simulink model "UDP_Send_Poi_2021b_openloop_joystick_2023"  (R2021b)
settings: Solver=FixedStepDiscrete  StartTime=0.0  StopTime=inf  FixedStep=0.05  RelTol=1e-3  EnableMultiTasking=on
undefined symbols (not defined in the file or in its folder): alpha_b_gain, DiscIntNeverNeededParam, Ts, z_l_gain
libraries: simulink x21, svdutilitieslib x10, raspberrypiNetworklib x2, dspstat3 x1
settings Model: SimulationMode=external  ExtModeTrigDuration=2  Creator=Sesh  LastModifiedBy=n7729
settings SolverCC: PositivePriorityOrder=on
settings OptimizationCC: EnhancedBackFolding=on  PassReuseOutputArgsAs=Individual arguments  ZeroExternalMemoryAtStartup=off  ZeroInternalMemoryAtStartup=off  MaxStackSize=64  OptimizeBlockOrder=speed  DifferentSizesBufferReuse=on  OptimizationCustomize=off  EfficientTunableParamExpr=on
settings DebuggingCC: ParameterTunabilityLossMsg=error  UnderSpecifiedDimensionMsg=warning
settings HardwareCC: ProdBitPerPointer=32  ProdBitPerSizeT=32  ProdBitPerPtrDiffT=32  ProdLargestAtomicInteger=Long  ProdLargestAtomicFloat=Double  ProdWordSize=32  ProdLongLongMode=on  ProdHWDeviceType=ARM Compatible->ARM Cortex
settings RTWCC: Description=Embedded Coder  SystemTargetFile=ert.tlc  HardwareBoard=Raspberry Pi  TLCOptions="-aInlineSetEventsForThisBaseRateFcn=TLC_FALSE -aSuppressMultiTaskScheduler=TLC_FALSE  -aRateBasedStepFcn=0"  TemplateMakefile=ert_default_tmf  Toolchain=GNU GCC Embedded Linux  BuildConfiguration=Faster Runs
settings CodeAppCC: ForceParamTrailComments=on  IgnoreCustomStorageClasses=off  OperatorAnnotations=on  SimulinkDataObjDesc=on  SFDataObjDesc=on  InsertBlockDesc=on
settings ERTTargetCC: SupportContinuousTime=on  SupportVariableSizeSignals=on  ExtMode=on  ExtModeTransport=2  ExtModeStaticAlloc=on  ExtModeMexFile=ext_xcp  ExtModeMexArgs='192.168.0.112' 0 17725  ExtModeIntrfLevel=Level2 - Open

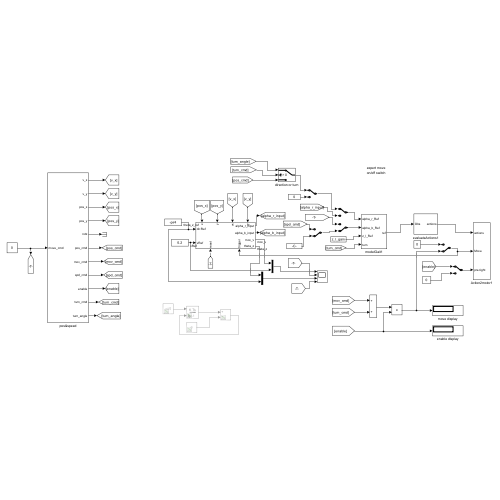
[thumbnail: Simulink's stored preview of the top-level diagram]
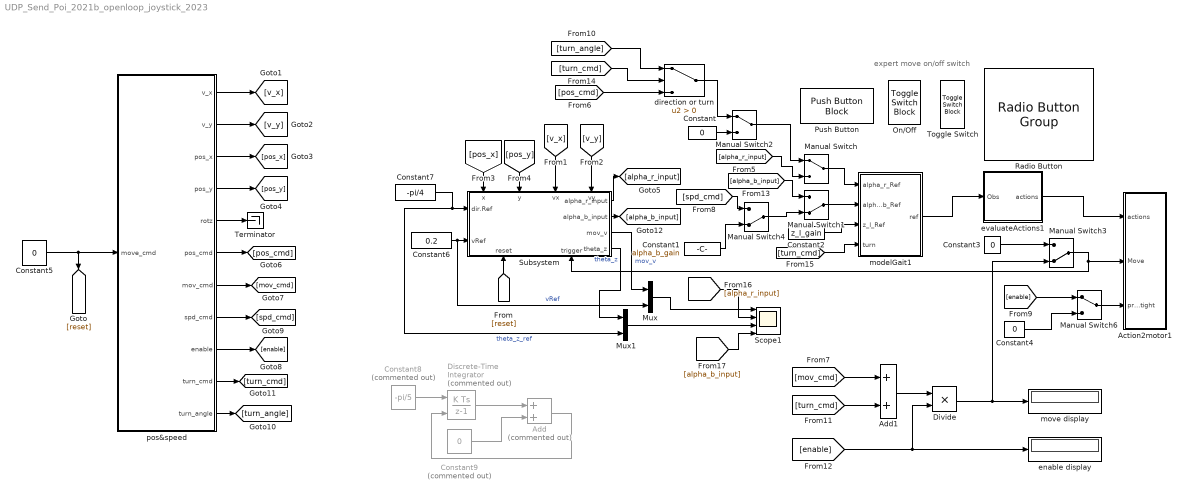
== system UDP_Send_Poi_2021b_openloop_joystick_2023 ==
  note: expert move
      | on/off switch
  Action2motor1 : Subsystem
  Add : Sum  Commented=on
  Add1 : Sum
  Constant{,3..5} (4 alike) : Constant  Value=0
  Constant1 : Constant  Value=alpha_b_gain
  Constant2 : Constant  Value=z_l_gain
  Constant6 : Constant  Value=0.2
  Constant7 : Constant  Value=-pi/4
  Constant8 : Constant  Commented=on  Value=-pi/5
  Constant9 : Constant  Commented=on  Value=0
  Discrete-Time Integrator : DiscreteIntegrator  Commented=on  ExternalReset=falling  SampleTime=Ts  ICPrevOutput=DiscIntNeverNeededParam  ICPrevScaledInput=DiscIntNeverNeededParam
  Divide : Product  Inputs=**
  Manual Switch : ManualSwitch
  Manual Switch1 : ManualSwitch  CurrentSetting=0
  Manual Switch2 : ManualSwitch
  Manual Switch3 : ManualSwitch  CurrentSetting=0
  Manual Switch4 : ManualSwitch  CurrentSetting=0
  Manual Switch6 : ManualSwitch
  Mux : Mux  Inputs=2
  Mux1 : Mux  Inputs=2
  On/Off : ToggleSwitchBlock  LabelPosition=Hide
      settings: Values={{'Off', 'On'}, [0 1]}
  Push Button : PushButtonBlock  ButtonText=reset_pos  OffValue=0.000000
  Radio Button : RadioButtonGroup  LabelPosition=Hide  SelectedLabel=front  ButtonGroupName=Direction
      settings: Values={{'front', 'back', 'left', 'right'}, [0 3.1416 1.5708 -1.5708]}
  Scope1 : Scope  NumInputPorts=4
  Subsystem : Subsystem
      settings: PortSchema="{\"entries\":[{\"content\":{\"sides\":[{\"content\":{\"connectorIds\":[\"In1\",\"In2\"]},\"type\":\"ConnectorPlacement.EquallySpacedRectSide\",\"uuid\":\"e0270cc0-a6da-4fa7-8263-2e1b5ac58467\"},{\"content\":{\"connectorIds\":[\"Out1\",\"Out2\",\"Out3\",\"Out4\"],\"side\":\"RIGHT\"},\"type\":\"ConnectorPlacement.EquallySpacedRectSide\",\"uuid\":\"f8f4d5ad-7603-452d-addd-169a876a6d80\"},{\"content\":{\"connectorIds\":[\"In3\",\"In4\",\"In5\",\"In6\"],\"side\":\"TOP\"},\"type\":\"ConnectorPlacement.EquallySpacedRectSide\",\"uuid\":\"9d841264-c6b3-49f6-8890-3bf3ae488520\"},{\"content\":{\"connectorIds\":[\"In7\",\"In8\"],\"side\":\"BOTTOM\"},\"type\":\"ConnectorPlacement.EquallySpacedRectSide\",\"uuid\":\"4462aa19-ad84-4319-8adf-52b01e042218\"}]},\"type\":\"ConnectorPlacement.EquallySpacedConnector\",\"uuid\":\"62223290-ed65-4858-a6ef-8a0888ac6d95\"}],\"packageUris\":[\"http://schema.mathworks.com/mf0/Connector/R2020b\"],\"version\":\"1.0\"}"
  Terminator : Terminator
  Toggle Switch : ToggleSwitchBlock  LabelPosition=Hide
      settings: Values={{'loose', 'tight'}, [0 1]}
  direction or turn : Switch  Criteria=u2 > Threshold
  enable display : Display
  evaluateActions1 : Subsystem
  modelGait1 : Subsystem
  move display : Display
  pos&speed : Subsystem
  wires:
  [turn_cmd] -> Add1/2
  Discrete-Time Integrator/1 -> Add/1
  Subsystem/2(alpha_b_input) -> [alpha_b_input]
  [alpha_r_input] -> Scope1/2
  Subsystem/1(alpha_r_input) -> [alpha_r_input]
  pos&speed/2(v_y) -> [v_y]
  modelGait1/1(ref) -> evaluateActions1/1(Obs)
  pos&speed/5(rotz) -> Terminator/1
  [mov_cmd] -> Add1/1
  Constant9/1 -> Add/2
  [spd_cmd] -> Manual Switch4/1
  Manual Switch3/1 -> Action2motor1/2(Move), Subsystem/8(trigger)
  pos&speed/9(enable) -> [enable]
  pos&speed/7(mov_cmd) -> [mov_cmd]
  pos&speed/1(v_x) -> [v_x]
  [pos_y] -> Subsystem/4(y)
  [alpha_r_input] -> Manual Switch/2
  [enable] -> Manual Switch6/1
  Subsystem/3(mov_v) -> Mux/1  "mov_v"
  pos&speed/11(turn_angle) -> [turn_angle]
  [pos_cmd] -> direction or turn/3
  [v_x] -> Subsystem/5(vx)
  pos&speed/3(pos_x) -> [pos_x]
  evaluateActions1/1(actions) -> Action2motor1/1(actions)
  Manual Switch1/1 -> modelGait1/2(alpha_b_Ref)
  pos&speed/6(pos_cmd) -> [pos_cmd]
  Constant7/1 -> Mux1/2, Subsystem/1(dir.Ref)  "theta_z_ref"
  [turn_cmd] -> modelGait1/4(turn)
  [v_y] -> Subsystem/6(vy)
  [alpha_b_input] -> Scope1/4
  pos&speed/10(turn_cmd) -> [turn_cmd]
  Divide/1 -> Manual Switch3/2, move display/1
  [turn_cmd] -> direction or turn/2
  Manual Switch4/1 -> Manual Switch1/2
  Constant3/1 -> Manual Switch3/1
  Constant8/1 -> Discrete-Time Integrator/1
  Subsystem/4(theta_z) -> Mux1/1  "theta_z"
  Constant2/1 -> modelGait1/3(z_l_Ref)
  [alpha_b_input] -> Manual Switch1/1
  Constant4/1 -> Manual Switch6/2
  Add1/1 -> Divide/1
  [reset] -> Subsystem/7(reset)
  pos&speed/8(spd_cmd) -> [spd_cmd]
  Manual Switch6/1 -> Action2motor1/3(pre-tight)
  Constant1/1 -> Manual Switch4/2
  Constant/1 -> Manual Switch2/2
  direction or turn/1 -> Manual Switch2/1
  pos&speed/4(pos_y) -> [pos_y]
  Manual Switch/1 -> modelGait1/1(alpha_r_Ref)
  [turn_angle] -> direction or turn/1
  Mux/1 -> Scope1/1
  Add/1 -> Discrete-Time Integrator/2
  [enable] -> enable display/1, Divide/2
  Constant6/1 -> Mux/2, Subsystem/2(vRef)  "vRef"
  Constant5/1 -> [reset], pos&speed/1(move_cmd)
  Mux1/1 -> Scope1/3
  Manual Switch2/1 -> Manual Switch/1
  [pos_x] -> Subsystem/3(x)

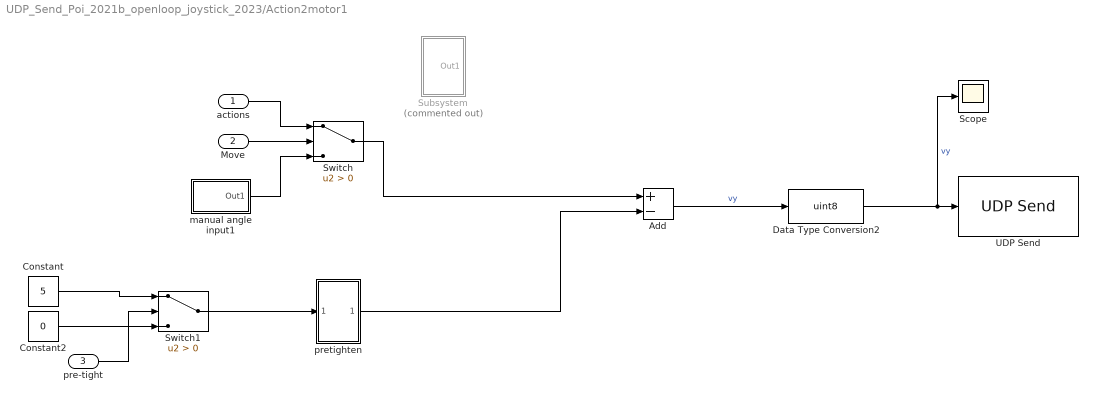
== system UDP_Send_Poi_2021b_openloop_joystick_2023/Action2motor1 ==
  actions : Inport
  Move : Inport  Port=2
  pre-tight : Inport  Port=3
  Add : Sum  Inputs=+-
  Constant : Constant  Value=5
  Constant2 : Constant  Value=0
  Data Type Conversion2 : DataTypeConversion  OutDataTypeStr=uint8
  Scope : Scope
  Subsystem : Subsystem  Commented=on
  Switch : Switch  Criteria=u2 > Threshold
  Switch1 : Switch  Criteria=u2 > Threshold
  UDP Send : raspberrypiNetworklib/UDP Send  remoteURL='0.0.0.0'  remotePort=8888  localURL='0.0.0.0'  localPortSource=Automatically determine  localPort=-1  sampletime=-1  blockPlatform=Raspberry Pi  separateLengthPort=0
      settings: SourceProductBaseCode=RASPPI
  manual angle input1 : Subsystem
  pretighten : Subsystem
  wires:
  actions/1 -> Switch/1
  manual angle input1/1(Out1) -> Switch/3
  pretighten/1(Out1) -> Add/2
  Switch/1 -> Add/1
  Switch1/1 -> pretighten/1(In1)
  Constant/1 -> Switch1/1
  Constant2/1 -> Switch1/3
  Data Type Conversion2/1 -> UDP Send/1, Scope/1  "vy"
  Add/1 -> Data Type Conversion2/1  "vy"
  Move/1 -> Switch/2
  pre-tight/1 -> Switch1/2

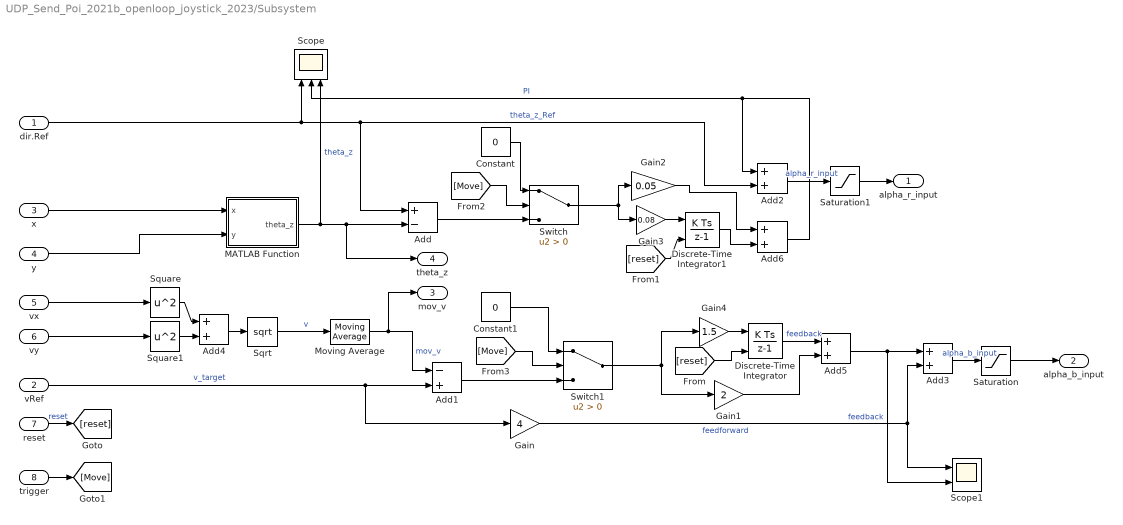
== system UDP_Send_Poi_2021b_openloop_joystick_2023/Subsystem ==
  dir.Ref : Inport
  vRef : Inport  Port=2
  x : Inport  Port=3
  y : Inport  Port=4
  vx : Inport  Port=5
  vy : Inport  Port=6
  reset : Inport  Port=7
  trigger : Inport  Port=8
  Add : Sum  Inputs=+-
  Add1 : Sum  Inputs=-+
  Add{2..6} (5 alike) : Sum
  Constant : Constant  Value=0
  Constant1 : Constant  Value=0
  Discrete-Time Integrator : DiscreteIntegrator  gainval=1  ExternalReset=rising  SampleTime=Ts  ICPrevOutput=DiscIntNeverNeededParam  ICPrevScaledInput=DiscIntNeverNeededParam
  Discrete-Time Integrator1 : DiscreteIntegrator  gainval=1  ExternalReset=rising  SampleTime=-1  ICPrevOutput=DiscIntNeverNeededParam  ICPrevScaledInput=DiscIntNeverNeededParam
  Gain : Gain  Gain=4
  Gain1 : Gain  Gain=2
  Gain2 : Gain  Gain=0.05
  Gain3 : Gain  Gain=0.08
  Gain4 : Gain  Gain=1.5
  MATLAB Function : MATLAB Function  TreatAsAtomicUnit=on
  Moving Average : dspstat3/Moving Average  Method=Sliding window  ForgettingFactorPort=off  SpecifyWindowLength=on  WindowLength=16  ForgettingFactor=0.9  SimulateUsing=Code generation
  Saturation : Saturate  UpperLimit=pi/3  LowerLimit=0
  Saturation1 : Saturate  UpperLimit=inf  LowerLimit=-inf
  Scope : Scope  NumInputPorts=3
  Scope1 : Scope  NumInputPorts=2
  Sqrt : Sqrt  SaturateOnIntegerOverflow=on
  Square : Math  Operator=square  SaturateOnIntegerOverflow=on
  Square1 : Math  Operator=square  SaturateOnIntegerOverflow=on
  Switch : Switch  Criteria=u2 > Threshold
  Switch1 : Switch  Criteria=u2 > Threshold
  alpha_r_input : Outport
  alpha_b_input : Outport  Port=2
  mov_v : Outport  Port=3
  theta_z : Outport  Port=4
  wires:
  Add4/1 -> Sqrt/1
  Square/1 -> Add4/1
  MATLAB Function/1(theta_z) -> Scope/3, Add/2, theta_z/1  "theta_z"
  vRef/1 -> Add1/2, Gain/1  "v_target"
  dir.Ref/1 -> Add2/2, Add/1, Scope/1  "theta_z_Ref"
  Square1/1 -> Add4/2
  Moving Average/1 -> Add1/1, mov_v/1  "mov_v"
  Add6/1 -> Add2/1, Scope/2  "PI"
  Add1/1 -> Switch1/3
  vy/1 -> Square1/1
  Sqrt/1 -> Moving Average/1  "v"
  y/1 -> MATLAB Function/2(y)
  Add2/1 -> Saturation1/1  "alpha_r_input"
  Add3/1 -> Saturation/1  "alpha_b_input"
  x/1 -> MATLAB Function/1(x)
  vx/1 -> Square/1
  Saturation/1 -> alpha_b_input/1
  Saturation1/1 -> alpha_r_input/1
  Switch/1 -> Gain3/1, Gain2/1
  Constant/1 -> Switch/1
  Add/1 -> Switch/3
  Switch1/1 -> Gain1/1, Gain4/1
  Constant1/1 -> Switch1/1
  Discrete-Time Integrator/1 -> Add5/1  "feedback"
  Gain1/1 -> Add5/2
  Discrete-Time Integrator1/1 -> Add6/2
  Gain2/1 -> Add6/1
  Gain3/1 -> Discrete-Time Integrator1/1
  Gain4/1 -> Discrete-Time Integrator/1
  reset/1 -> [reset]  "reset"
  [reset] -> Discrete-Time Integrator/2
  [reset] -> Discrete-Time Integrator1/2
  trigger/1 -> [Move]
  [Move] -> Switch/2
  [Move] -> Switch1/2
  Add5/1 -> Scope1/2, Add3/1  "feedback"
  Gain/1 -> Scope1/1, Add3/2  "feedforward"

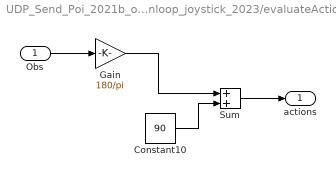
== system UDP_Send_Poi_2021b_openloop_joystick_2023/evaluateActions1 ==
  Obs : Inport
  Constant10 : Constant  Value=90
  Gain : Gain  Gain=180/pi
  Sum : Sum
  actions : Outport  OutDataTypeStr=double
  wires:
  Gain/1 -> Sum/1
  Sum/1 -> actions/1
  Obs/1 -> Gain/1
  Constant10/1 -> Sum/2

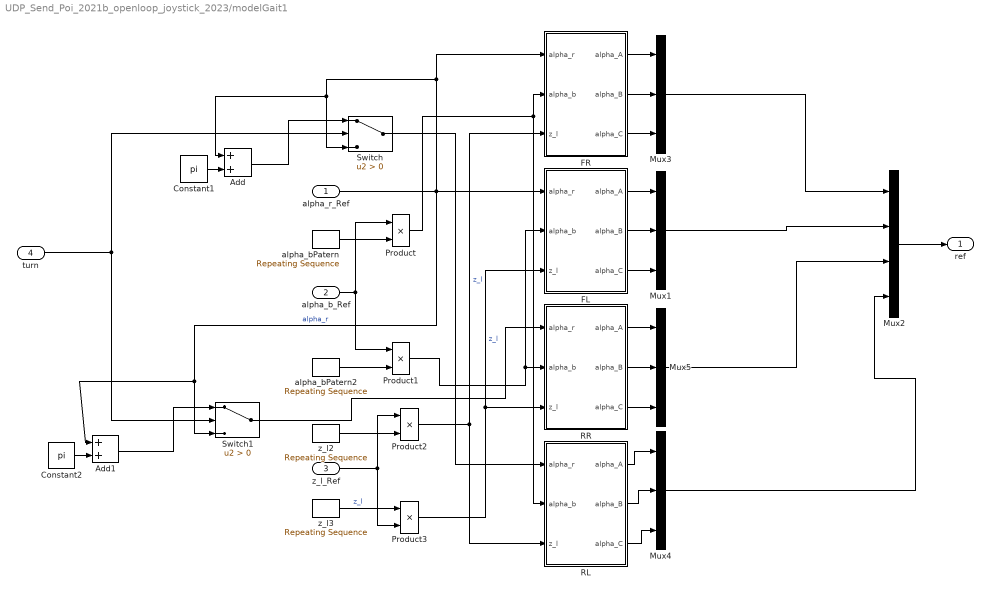
== system UDP_Send_Poi_2021b_openloop_joystick_2023/modelGait1 ==
  alpha_r_Ref : Inport
  alpha_b_Ref : Inport  Port=2
  z_l_Ref : Inport  Port=3
  turn : Inport  Port=4
  Add : Sum
  Add1 : Sum
  Constant1 : Constant  Value=pi
  Constant2 : Constant  Value=pi
  FL : MATLAB Function  TreatAsAtomicUnit=on
  FR : MATLAB Function  TreatAsAtomicUnit=on
  Mux{1,3..5} (4 alike) : Mux  Inputs=3
  Mux2 : Mux
  Product{,1..3} (4 alike) : Product
  RL : MATLAB Function  TreatAsAtomicUnit=on
  RR : MATLAB Function  TreatAsAtomicUnit=on
  Switch : Switch  Criteria=u2 > Threshold
  Switch1 : Switch  Criteria=u2 > Threshold
  alpha_bPatern : simulink/Sources/Repeating Sequence  rep_seq_t=[0 0.2 0.4 0.6 0.8]  rep_seq_y=[0 1 0 -1 0]
  alpha_bPatern2 : simulink/Sources/Repeating Sequence  rep_seq_t=[0 0.2 0.4 0.6 0.8]  rep_seq_y=[0 -1 0 1 0]
  z_l2 : simulink/Sources/Repeating Sequence  rep_seq_t=[0 0.2 0.4 0.6 0.8]  rep_seq_y=[0 0 1 0 0]
  z_l3 : simulink/Sources/Repeating Sequence  rep_seq_t=[0 0.2 0.4 0.6 0.8]  rep_seq_y=[1 0 0 0 1]
  ref : Outport
  wires:
  FR/1(alpha_A) -> Mux3/1
  Product2/1 -> FR/3(z_l), RL/3(z_l)  "z_l"
  FR/2(alpha_B) -> Mux3/2
  FR/3(alpha_C) -> Mux3/3
  Product3/1 -> FL/3(z_l), RR/3(z_l)  "z_l"
  FL/3(alpha_C) -> Mux1/3
  alpha_r_Ref/1 -> Switch1/3, Add1/1, FL/1(alpha_r), FR/1(alpha_r), Switch/3, Add/1  "alpha_r"
  FL/2(alpha_B) -> Mux1/2
  FL/1(alpha_A) -> Mux1/1
  alpha_bPatern/1 -> Product/2
  alpha_b_Ref/1 -> Product/1, Product1/1
  Product/1 -> RL/2(alpha_b), FR/2(alpha_b)
  alpha_bPatern2/1 -> Product1/2
  Product1/1 -> FL/2(alpha_b), RR/2(alpha_b)
  z_l2/1 -> Product2/2
  z_l_Ref/1 -> Product3/2, Product2/1
  z_l3/1 -> Product3/1  "z_l"
  RL/3(alpha_C) -> Mux4/3
  RL/2(alpha_B) -> Mux4/2
  RL/1(alpha_A) -> Mux4/1
  Mux3/1 -> Mux2/1
  RR/3(alpha_C) -> Mux5/3
  RR/1(alpha_A) -> Mux5/1
  RR/2(alpha_B) -> Mux5/2
  Switch/1 -> RL/1(alpha_r)
  Constant1/1 -> Add/2
  Add/1 -> Switch/1
  Switch1/1 -> RR/1(alpha_r)
  Add1/1 -> Switch1/1
  Constant2/1 -> Add1/2
  turn/1 -> Switch1/2, Switch/2
  Mux2/1 -> ref/1
  Mux1/1 -> Mux2/2
  Mux4/1 -> Mux2/4
  Mux5/1 -> Mux2/3

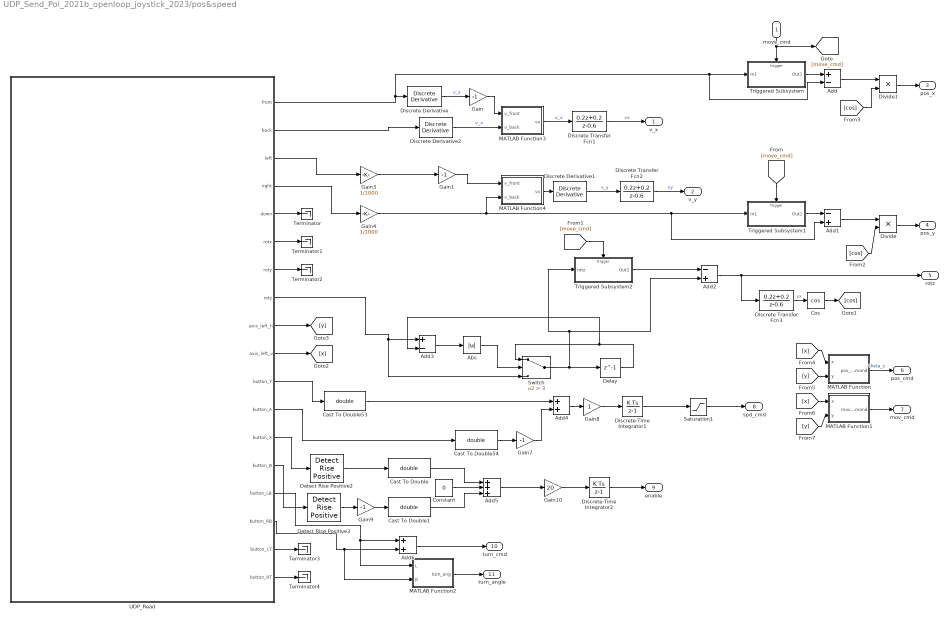
== system UDP_Send_Poi_2021b_openloop_joystick_2023/pos&speed ==
  move_cmd : Inport
  Abs : Abs
  Add : Sum  Inputs=+-
  Add1 : Sum  Inputs=-+
  Add2 : Sum  Inputs=-+
  Add3 : Sum  Inputs=+-
  Add4 : Sum
  Add5 : Sum  Inputs=+++
  Add6 : Sum
  Cast To Double{,1,53..54} (4 alike) : DataTypeConversion  OutDataTypeStr=double
  Constant : Constant  Value=0
  Cos : Trigonometry  Operator=cos
  Delay : Delay  DelayLength=1
  Detect Rise Positive2 : simulink/Logic and Bit Operations/Detect Rise Positive  vinit=0  OutDataTypeStr=boolean
  Detect Rise Positive3 : simulink/Logic and Bit Operations/Detect Rise Positive  vinit=0  OutDataTypeStr=boolean
  Discrete Transfer Fcn1 : DiscreteTransferFcn  Numerator=[0.2 0.2]  Denominator=[1 -0.6]
  Discrete Transfer Fcn2 : DiscreteTransferFcn  Numerator=[0.2 0.2]  Denominator=[1 -0.6]
  Discrete Transfer Fcn3 : DiscreteTransferFcn  Numerator=[0.2 0.2]  Denominator=[1 -0.6]
  Discrete Derivative : simulink/Discrete/Discrete Derivative  gainval=1.0  ICPrevScaledInput=0.0  OutMin=[]  OutMax=[]  OutDataType=fixdt(1, 16)  OutScaling=2^-10  DoSatur=off
  Discrete Derivative1 : simulink/Discrete/Discrete Derivative  gainval=1.0  ICPrevScaledInput=0.0  OutMin=[]  OutMax=[]  OutDataType=fixdt(1, 16)  OutScaling=2^-10  DoSatur=off
  Discrete Derivative2 : simulink/Discrete/Discrete Derivative  gainval=1.0  ICPrevScaledInput=0.0  OutMin=[]  OutMax=[]  OutDataType=fixdt(1, 16)  OutScaling=2^-10  DoSatur=off
  Discrete-Time Integrator1 : DiscreteIntegrator  InitialCondition=pi/12  SampleTime=-1  LimitOutput=on  UpperSaturationLimit=pi/4  LowerSaturationLimit=pi/12  ICPrevOutput=DiscIntNeverNeededParam  ICPrevScaledInput=DiscIntNeverNeededParam
  Discrete-Time Integrator2 : DiscreteIntegrator  SampleTime=-1  LimitOutput=on  UpperSaturationLimit=1  LowerSaturationLimit=0  ICPrevOutput=DiscIntNeverNeededParam  ICPrevScaledInput=DiscIntNeverNeededParam
  Divide : Product  Inputs=**
  Divide1 : Product  Inputs=**
  Gain{,1,7,9} (4 alike) : Gain  Gain=-1
  Gain10 : Gain  Gain=20
  Gain3 : Gain  Gain=1/1000
  Gain4 : Gain  Gain=1/1000
  Gain8 : Gain
  MATLAB Function : MATLAB Function  TreatAsAtomicUnit=on
  MATLAB Function1 : MATLAB Function  TreatAsAtomicUnit=on
  MATLAB Function2 : MATLAB Function  TreatAsAtomicUnit=on
  MATLAB Function3 : MATLAB Function  TreatAsAtomicUnit=on
  MATLAB Function4 : MATLAB Function  TreatAsAtomicUnit=on
  Saturation1 : Saturate  UpperLimit=pi/4  LowerLimit=pi/12
  Switch : Switch  Criteria=u2 > Threshold  Threshold=3
  Terminator{,1..4} (5 alike) : Terminator
  Triggered Subsystem : Subsystem  TreatAsAtomicUnit=on
  Triggered Subsystem1 : Subsystem  TreatAsAtomicUnit=on
  Triggered Subsystem2 : Subsystem  TreatAsAtomicUnit=on
  UDP_Read : Subsystem
  v_x : Outport
  v_y : Outport  Port=2
  pos_x : Outport  Port=3
  pos_y : Outport  Port=4
  rotz : Outport  Port=5
  pos_cmd : Outport  Port=6
  mov_cmd : Outport  Port=7
  spd_cmd : Outport  Port=8
  enable : Outport  Port=9
  turn_cmd : Outport  Port=10
  turn_angle : Outport  Port=11
  wires:
  Gain1/1 -> MATLAB Function4/1(v_front)
  UDP_Read/4(right) -> Gain4/1
  UDP_Read/1(front) -> Discrete Derivative/1, Triggered Subsystem/1(In1), Add/2
  Gain/1 -> MATLAB Function3/1(v_front)
  Gain3/1 -> Gain1/1
  UDP_Read/5(down) -> Terminator/1
  Discrete Derivative1/1 -> Discrete Transfer Fcn2/1  "v_y"
  move_cmd/1 -> Triggered Subsystem/Trigger, [move_cmd]
  Triggered Subsystem/1(Out1) -> Add/1
  Triggered Subsystem1/1(Out1) -> Add1/1
  MATLAB Function4/1(vx) -> Discrete Derivative1/1
  UDP_Read/3(left) -> Gain3/1
  UDP_Read/6(rotx) -> Terminator1/1
  UDP_Read/7(roty) -> Terminator2/1
  Triggered Subsystem2/1(Out1) -> Add2/1
  Add2/1 -> rotz/1, Discrete Transfer Fcn3/1
  Add1/1 -> Divide/1
  Divide/1 -> pos_y/1
  Divide1/1 -> pos_x/1
  Add/1 -> Divide1/1
  Gain4/1 -> MATLAB Function4/2(v_back), Add1/2, Triggered Subsystem1/1(In1)
  Discrete Transfer Fcn1/1 -> v_x/1  "vx"
  Discrete Transfer Fcn2/1 -> v_y/1  "vy"
  Discrete Transfer Fcn3/1 -> Cos/1  "vx"
  UDP_Read/8(rotz) -> Switch/3, Add3/1
  Add3/1 -> Abs/1
  Abs/1 -> Switch/2
  Switch/1 -> Triggered Subsystem2/1(rotz), Add2/2, Delay/1
  Delay/1 -> Add3/2, Switch/1
  MATLAB Function/1(pos_command) -> pos_cmd/1  "theta_z"
  MATLAB Function1/1(move_command) -> mov_cmd/1
  Gain8/1 -> Discrete-Time Integrator1/1
  Discrete-Time Integrator1/1 -> Saturation1/1
  Cast To Double53/1 -> Add4/1
  Gain7/1 -> Add4/2
  UDP_Read/12(button_A) -> Cast To Double54/1
  Add4/1 -> Gain8/1
  Cast To Double54/1 -> Gain7/1
  Saturation1/1 -> spd_cmd/1
  UDP_Read/13(button_X) -> Detect Rise Positive2/1
  UDP_Read/14(button_B) -> Detect Rise Positive3/1
  Detect Rise Positive3/1 -> Gain9/1
  Detect Rise Positive2/1 -> Cast To Double/1
  Gain9/1 -> Cast To Double1/1
  Add5/1 -> Gain10/1
  Discrete-Time Integrator2/1 -> enable/1
  Cast To Double/1 -> Add5/1
  UDP_Read/11(button_Y) -> Cast To Double53/1
  Gain10/1 -> Discrete-Time Integrator2/1
  UDP_Read/15(button_LB) -> MATLAB Function2/1(L), Add6/1
  UDP_Read/16(button_RB) -> MATLAB Function2/2(R), Add6/2
  Add6/1 -> turn_cmd/1
  MATLAB Function2/1(turn_ang) -> turn_angle/1
  [move_cmd] -> Triggered Subsystem1/Trigger
  [move_cmd] -> Triggered Subsystem2/Trigger
  Cos/1 -> [cos]
  [cos] -> Divide1/2
  [cos] -> Divide/2
  UDP_Read/9(axis_left_h) -> [y]
  [x] -> MATLAB Function/1(x)
  [x] -> MATLAB Function1/1(x)
  UDP_Read/10(axis_left_v) -> [x]
  [y] -> MATLAB Function1/2(y)
  [y] -> MATLAB Function/2(y)
  Constant/1 -> Add5/2
  Cast To Double1/1 -> Add5/3
  UDP_Read/17(button_LT) -> Terminator3/1
  UDP_Read/18(button_RT) -> Terminator4/1
  Discrete Derivative/1 -> Gain/1  "v_x"
  Discrete Derivative2/1 -> MATLAB Function3/2(v_back)  "v_x"
  MATLAB Function3/1(vx) -> Discrete Transfer Fcn1/1  "v_x"
  UDP_Read/2(back) -> Discrete Derivative2/1

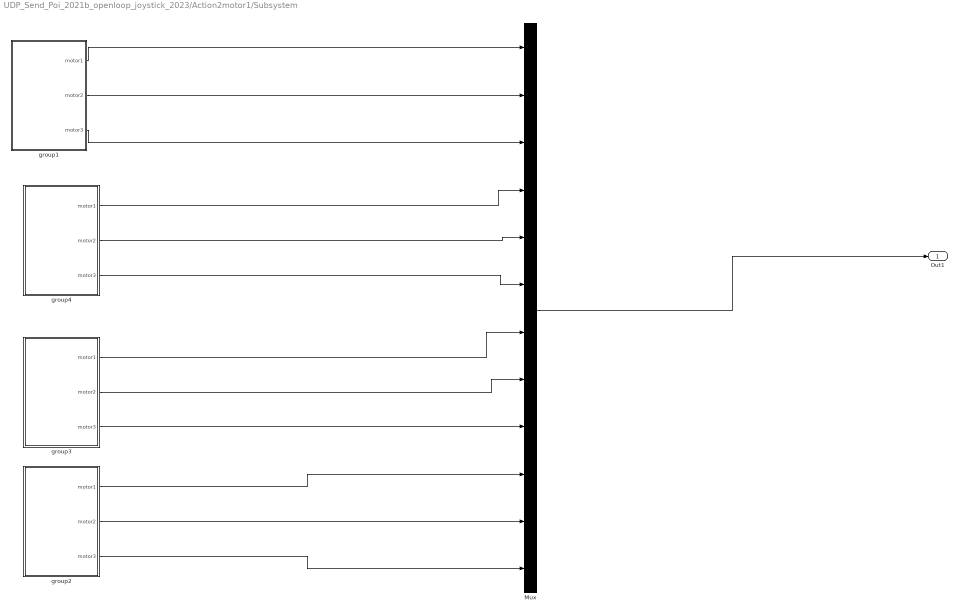
== system UDP_Send_Poi_2021b_openloop_joystick_2023/Action2motor1/Subsystem ==
  Mux : Mux  Inputs=12
  group1 : Subsystem
  group2 : Subsystem
  group3 : Subsystem
  group4 : Subsystem
  Out1 : Outport
  wires:
  group1/1(motor1) -> Mux/1
  group2/1(motor1) -> Mux/10
  group2/3(motor3) -> Mux/12
  group4/2(motor2) -> Mux/5
  group3/2(motor2) -> Mux/8
  group4/1(motor1) -> Mux/4
  group1/3(motor3) -> Mux/3
  group2/2(motor2) -> Mux/11
  group1/2(motor2) -> Mux/2
  Mux/1 -> Out1/1
  group3/1(motor1) -> Mux/7
  group3/3(motor3) -> Mux/9
  group4/3(motor3) -> Mux/6

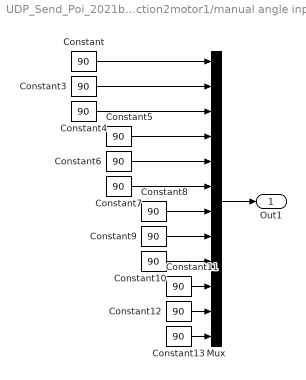
== system UDP_Send_Poi_2021b_openloop_joystick_2023/Action2motor1/manual angle input1 ==
  Constant{,3..13} (12 alike) : Constant  Value=90  SampleTime=-1
  Mux : Mux  Inputs=12
  Out1 : Outport
  wires:
  Constant3/1 -> Mux/2
  Constant11/1 -> Mux/10
  Constant9/1 -> Mux/8
  Constant8/1 -> Mux/7
  Constant/1 -> Mux/1
  Constant4/1 -> Mux/3
  Constant10/1 -> Mux/9
  Constant5/1 -> Mux/4
  Constant7/1 -> Mux/6
  Constant13/1 -> Mux/12
  Constant12/1 -> Mux/11
  Constant6/1 -> Mux/5
  Mux/1 -> Out1/1

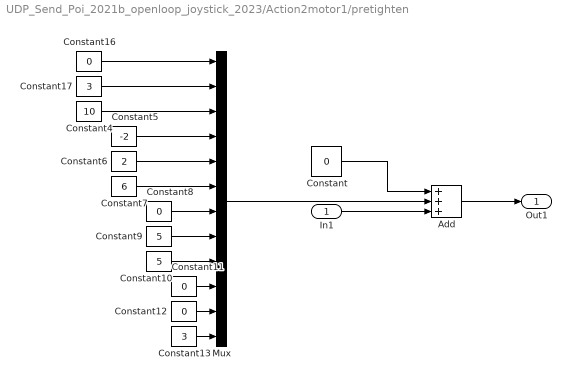
== system UDP_Send_Poi_2021b_openloop_joystick_2023/Action2motor1/pretighten ==
  In1 : Inport
  Add : Sum  Inputs=+++
  Constant : Constant  Value=0
  Constant10 : Constant  Value=5  SampleTime=-1
  Constant{8,11..12,16} (4 alike) : Constant  Value=0  SampleTime=-1
  Constant13 : Constant  Value=3  SampleTime=-1
  Constant17 : Constant  Value=3  SampleTime=-1
  Constant4 : Constant  Value=10  SampleTime=-1
  Constant5 : Constant  Value=-2  SampleTime=-1
  Constant6 : Constant  Value=2  SampleTime=-1
  Constant7 : Constant  Value=6  SampleTime=-1
  Constant9 : Constant  Value=5  SampleTime=-1
  Mux : Mux  Inputs=12
  Out1 : Outport
  wires:
  Constant12/1 -> Mux/11
  Constant6/1 -> Mux/5
  Constant9/1 -> Mux/8
  Constant4/1 -> Mux/3
  Constant13/1 -> Mux/12
  Constant7/1 -> Mux/6
  Constant5/1 -> Mux/4
  Mux/1 -> Add/2
  Constant10/1 -> Mux/9
  Constant8/1 -> Mux/7
  Constant11/1 -> Mux/10
  Constant17/1 -> Mux/2
  Constant/1 -> Add/1
  Constant16/1 -> Mux/1
  Add/1 -> Out1/1
  In1/1 -> Add/3

== system UDP_Send_Poi_2021b_openloop_joystick_2023/pos&speed/Triggered Subsystem ==
  In1 : Inport
  Trigger : TriggerPort  VariantControl=(inherit)
  Out1 : Outport
  wires:
  In1/1 -> Out1/1

== system UDP_Send_Poi_2021b_openloop_joystick_2023/pos&speed/Triggered Subsystem1 ==
  In1 : Inport
  Trigger : TriggerPort  VariantControl=(inherit)
  Out1 : Outport
  wires:
  In1/1 -> Out1/1

== system UDP_Send_Poi_2021b_openloop_joystick_2023/pos&speed/Triggered Subsystem2 ==
  rotz : Inport
  Trigger : TriggerPort  VariantControl=(inherit)
  Out1 : Outport
  wires:
  rotz/1 -> Out1/1

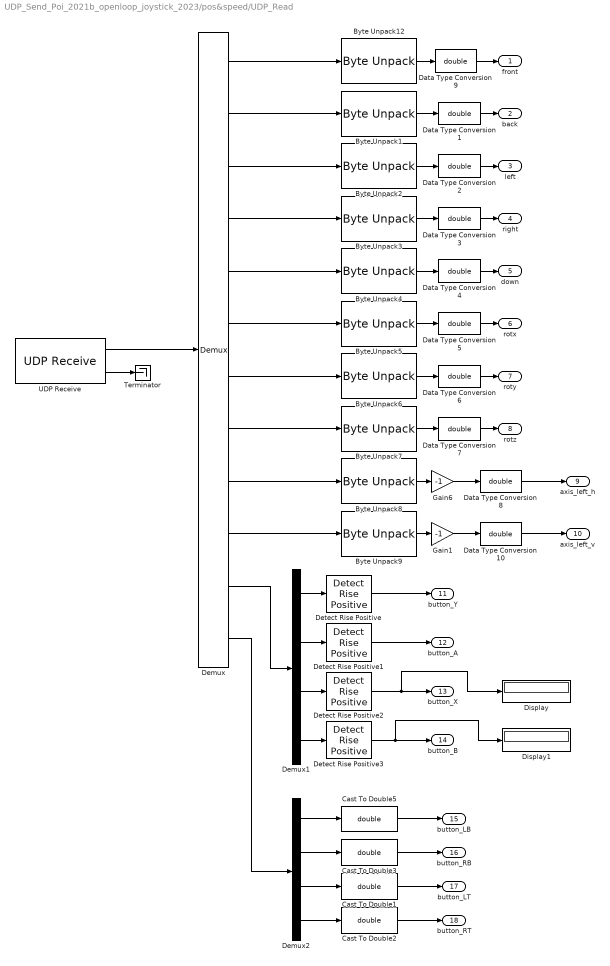
== system UDP_Send_Poi_2021b_openloop_joystick_2023/pos&speed/UDP_Read ==
  Byte Unpack{1..9,12} (10 alike) : svdutilitieslib/Byte Unpack  dimensions={[1]}  datatypes={'single'}  byteAlign=1  blockPlatform=arduinoert
      settings: SourceProductBaseCode=ANDROID,ARDUINO,ML_ARDUINO,ECCORTEXA,ECCORTEXR,SC_BEAGLEBONE_BLUE,EC_FREEDOM_BOARD,EC_FRDM_K64F,INTEL_BLOCKSET,MICROBIT,NUCLEO,NVIDIA,PX4AUTOPILOTS,RASPPIIO,STMICRODIS,TIC2000,XILINX_BLOCKSET
  Cast To Double{1..3,5} (4 alike) : DataTypeConversion  OutDataTypeStr=double
  Data Type Conversion{1..10} (10 alike) : DataTypeConversion  OutDataTypeStr=double
  Demux : Demux  Outputs=12
  Demux1 : Demux
  Demux2 : Demux
  Detect Rise Positive{,1..3} (4 alike) : simulink/Logic and Bit Operations/Detect Rise Positive  vinit=0  OutDataTypeStr=boolean
  Display : Display
  Display1 : Display
  Gain1 : Gain  Gain=-1
  Gain6 : Gain  Gain=-1
  Terminator : Terminator
  UDP Receive : raspberrypiNetworklib/UDP Receive  localURL='0.0.0.0'  localPort=6666  remoteURL='0.0.0.0'  remotePort=-1  recvBufferSize=8192  signalDatatype=uint8  dims=48  isVarSize=off  showBlockingTime=off  blockingTime=0  sampletime=-1  blockPlatform=Raspberry Pi
      settings: SourceProductBaseCode=RASPPI
  front : Outport
  back : Outport  Port=2
  left : Outport  Port=3
  right : Outport  Port=4
  down : Outport  Port=5
  rotx : Outport  Port=6
  roty : Outport  Port=7
  rotz : Outport  Port=8
  axis_left_h : Outport  Port=9
  axis_left_v : Outport  Port=10
  button_Y : Outport  Port=11
  button_A : Outport  Port=12
  button_X : Outport  Port=13
  button_B : Outport  Port=14
  button_LB : Outport  Port=15
  button_RB : Outport  Port=16
  button_LT : Outport  Port=17
  button_RT : Outport  Port=18
  wires:
  Byte Unpack3/1 -> Data Type Conversion3/1
  Byte Unpack12/1 -> Data Type Conversion9/1
  Demux/3 -> Byte Unpack2/1
  Demux/2 -> Byte Unpack1/1
  Demux/5 -> Byte Unpack4/1
  UDP Receive/2 -> Terminator/1
  Byte Unpack4/1 -> Data Type Conversion4/1
  Demux/1 -> Byte Unpack12/1
  Byte Unpack1/1 -> Data Type Conversion1/1
  Byte Unpack2/1 -> Data Type Conversion2/1
  Demux/4 -> Byte Unpack3/1
  Demux/6 -> Byte Unpack5/1
  Demux/7 -> Byte Unpack6/1
  Demux/8 -> Byte Unpack7/1
  Byte Unpack5/1 -> Data Type Conversion5/1
  Byte Unpack6/1 -> Data Type Conversion6/1
  Byte Unpack7/1 -> Data Type Conversion7/1
  Demux/9 -> Byte Unpack8/1
  Demux/10 -> Byte Unpack9/1
  Byte Unpack8/1 -> Gain6/1
  Byte Unpack9/1 -> Gain1/1
  Detect Rise Positive/1 -> button_Y/1
  Demux1/2 -> Detect Rise Positive1/1
  Demux1/3 -> Detect Rise Positive2/1
  Demux1/4 -> Detect Rise Positive3/1
  Demux/11 -> Demux1/1
  Demux1/1 -> Detect Rise Positive/1
  Demux2/1 -> Cast To Double5/1
  Demux2/3 -> Cast To Double1/1
  Demux/12 -> Demux2/1
  Demux2/2 -> Cast To Double3/1
  Demux2/4 -> Cast To Double2/1
  Cast To Double5/1 -> button_LB/1
  Cast To Double3/1 -> button_RB/1
  Data Type Conversion9/1 -> front/1
  Data Type Conversion1/1 -> back/1
  Data Type Conversion2/1 -> left/1
  Data Type Conversion3/1 -> right/1
  Data Type Conversion4/1 -> down/1
  Data Type Conversion5/1 -> rotx/1
  Data Type Conversion6/1 -> roty/1
  Data Type Conversion7/1 -> rotz/1
  Gain6/1 -> Data Type Conversion8/1
  Gain1/1 -> Data Type Conversion10/1
  Data Type Conversion8/1 -> axis_left_h/1
  Data Type Conversion10/1 -> axis_left_v/1
  Detect Rise Positive1/1 -> button_A/1
  Detect Rise Positive2/1 -> Display/1, button_X/1
  Detect Rise Positive3/1 -> Display1/1, button_B/1
  Cast To Double1/1 -> button_LT/1
  Cast To Double2/1 -> button_RT/1
  UDP Receive/1 -> Demux/1

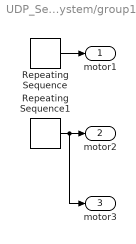
== system UDP_Send_Poi_2021b_openloop_joystick_2023/Action2motor1/Subsystem/group1 ==
  Repeating Sequence : simulink/Sources/Repeating Sequence  rep_seq_t=out.G1M1Data.time  rep_seq_y=out.G1M1Data.signals.values
  Repeating Sequence1 : simulink/Sources/Repeating Sequence  rep_seq_t=out.G1M23Data.time  rep_seq_y=out.G1M23Data.signals.values
  motor1 : Outport  VectorParamsAs1DForOutWhenUnconnected=off
  motor2 : Outport  Port=2  VectorParamsAs1DForOutWhenUnconnected=off
  motor3 : Outport  Port=3  VectorParamsAs1DForOutWhenUnconnected=off
  wires:
  Repeating Sequence1/1 -> motor3/1, motor2/1
  Repeating Sequence/1 -> motor1/1

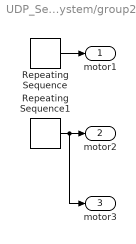
== system UDP_Send_Poi_2021b_openloop_joystick_2023/Action2motor1/Subsystem/group2 ==
  Repeating Sequence : simulink/Sources/Repeating Sequence  rep_seq_t=out.G1M1Data.time  rep_seq_y=out.G1M1Data.signals.values
  Repeating Sequence1 : simulink/Sources/Repeating Sequence  rep_seq_t=out.G1M23Data.time  rep_seq_y=out.G1M23Data.signals.values
  motor1 : Outport  VectorParamsAs1DForOutWhenUnconnected=off
  motor2 : Outport  Port=2  VectorParamsAs1DForOutWhenUnconnected=off
  motor3 : Outport  Port=3  VectorParamsAs1DForOutWhenUnconnected=off
  wires:
  Repeating Sequence1/1 -> motor3/1, motor2/1
  Repeating Sequence/1 -> motor1/1

== system UDP_Send_Poi_2021b_openloop_joystick_2023/Action2motor1/Subsystem/group3 ==
  Repeating Sequence : simulink/Sources/Repeating Sequence  rep_seq_t=out.G3M1Data1.time  rep_seq_y=out.G3M1Data1.signals.values
  Repeating Sequence1 : simulink/Sources/Repeating Sequence  rep_seq_t=out.G3M23Data.time  rep_seq_y=out.G3M23Data.signals.values
  motor1 : Outport  VectorParamsAs1DForOutWhenUnconnected=off
  motor2 : Outport  Port=2  VectorParamsAs1DForOutWhenUnconnected=off
  motor3 : Outport  Port=3  VectorParamsAs1DForOutWhenUnconnected=off
  wires:
  Repeating Sequence1/1 -> motor3/1, motor2/1
  Repeating Sequence/1 -> motor1/1

== system UDP_Send_Poi_2021b_openloop_joystick_2023/Action2motor1/Subsystem/group4 ==
  Repeating Sequence : simulink/Sources/Repeating Sequence  rep_seq_t=out.G3M1Data1.time  rep_seq_y=out.G3M1Data1.signals.values
  Repeating Sequence1 : simulink/Sources/Repeating Sequence  rep_seq_t=out.G3M23Data.time  rep_seq_y=out.G3M23Data.signals.values
  motor1 : Outport  VectorParamsAs1DForOutWhenUnconnected=off
  motor2 : Outport  Port=2  VectorParamsAs1DForOutWhenUnconnected=off
  motor3 : Outport  Port=3  VectorParamsAs1DForOutWhenUnconnected=off
  wires:
  Repeating Sequence1/1 -> motor3/1, motor2/1
  Repeating Sequence/1 -> motor1/1

== matlab function UDP_Send_Poi_2021b_openloop_joystick_2023/pos&speed/MATLAB Function ==
  data: x input; pos_command output; y input
function pos_command = fcn(x, y)
if y >=-0.5 && y<= 0.5 && x >= -0.5 && x <= 0.5
    pos_command = 0; % no move, joystick in center
else
if y == 0 && x >= 0
    pos_command = 0; % joystick up, move forward
elseif y == 0 && x < 0
    pos_command = pi; % joystick down, move backward
else
    pos_command = atan(y/x); % o.w., calculate the turn angle
end

% limit the angle calculation
if x<0 && y<0
    pos_command = pos_command - pi;
end
if x<0 && y>0
    pos_command = pos_command + pi;
end

if pos_command < -pi*0.99
    pos_command = pos_command + 2*pi;
end
end

== matlab function UDP_Send_Poi_2021b_openloop_joystick_2023/pos&speed/MATLAB Function1 ==
  data: x input; move_command output; y input
function move_command = mov_cmd(x,y)
if y >=-0.5 && y<= 0.5 && x >= -0.5 && x <= 0.5
    move_command = 0;
else
    move_command =1;
end

== matlab function UDP_Send_Poi_2021b_openloop_joystick_2023/pos&speed/MATLAB Function2 ==
  data: L input; turn_ang output; R input
function turn_ang = turn_angle(L,R)

if L == 1 && R == 0
    turn_ang = pi/2;
elseif L == 0 && R == 1
    turn_ang = -pi/2;
else
    turn_ang = 0;
end

== matlab function UDP_Send_Poi_2021b_openloop_joystick_2023/Subsystem/MATLAB Function ==
  data: x input; theta_z output; y input
function theta_z = fcn(x, y)

if y == 0 && x >= 0
    theta_z = 0;
elseif y == 0 && x < 0
    theta_z = pi;
else
    theta_z = atan(y/x);
end

if x<0 && y<0
    theta_z = theta_z - pi;
end
if x<0 && y>0
    theta_z = theta_z + pi;
end

if theta_z < -pi*0.99
    theta_z = theta_z + 2*pi;
end

== matlab function UDP_Send_Poi_2021b_openloop_joystick_2023/pos&speed/MATLAB Function3 ==
  data: v_front input; vx output; v_back input
function vx = fcn(v_front, v_back)

if abs(v_front) >= 400 || abs(v_back) < 400
    vx = v_back;
elseif abs(v_back) >= 400 || abs(v_front) < 400
    vx = v_front;
else
    vx = (v_back + v_front)/2;
end

== matlab function UDP_Send_Poi_2021b_openloop_joystick_2023/pos&speed/MATLAB Function4 ==
  data: v_front input; vx output; v_back input
function vx = fcn(v_front, v_back)

if abs(v_front) >= 400 || abs(v_back) < 400
    vx = v_back;
elseif abs(v_back) >= 400 || abs(v_front) < 400
    vx = v_front;
else
    vx = (v_back + v_front)/2;
end

== matlab function UDP_Send_Poi_2021b_openloop_joystick_2023/modelGait1/FR ==
  data: alpha_r input; alpha_A output; alpha_b input; z_l input; alpha_B output; alpha_C output
function [alpha_A, alpha_B, alpha_C]= fcn(alpha_r, alpha_b, z_l)

L_disk = 0.02944;% Disk side length (m)
R_spool = 0.021;
R_w = L_disk/sqrt(3);

alpha_A = -(-R_w*alpha_b*cos(-alpha_r)+z_l)/R_spool;
alpha_B = -(-R_w*alpha_b*cos(-alpha_r+2*pi/3)+z_l)/R_spool;
alpha_C = -(-R_w*alpha_b*cos(-alpha_r+4*pi/3)+z_l)/R_spool;

== matlab function UDP_Send_Poi_2021b_openloop_joystick_2023/modelGait1/FL ==
  data: alpha_r input; alpha_A output; alpha_b input; z_l input; alpha_B output; alpha_C output
function [alpha_A, alpha_B, alpha_C]= fcn(alpha_r, alpha_b, z_l)

L_disk = 0.02944;% Disk side length (m)
R_spool = 0.021;
R_w = L_disk/sqrt(3);

alpha_A = -(-R_w*alpha_b*cos(-alpha_r)+z_l)/R_spool;
alpha_B = -(-R_w*alpha_b*cos(-alpha_r+2*pi/3)+z_l)/R_spool;
alpha_C = -(-R_w*alpha_b*cos(-alpha_r+4*pi/3)+z_l)/R_spool;

== matlab function UDP_Send_Poi_2021b_openloop_joystick_2023/modelGait1/RL ==
  data: alpha_r input; alpha_A output; alpha_b input; z_l input; alpha_B output; alpha_C output
function [alpha_A, alpha_B, alpha_C]= fcn(alpha_r, alpha_b, z_l)

L_disk = 0.02944;% Disk side length (m)
R_spool = 0.021;
R_w = L_disk/sqrt(3);

alpha_A = -(-R_w*alpha_b*cos(-alpha_r)+z_l)/R_spool;
alpha_B = -(-R_w*alpha_b*cos(-alpha_r+2*pi/3)+z_l)/R_spool;
alpha_C = -(-R_w*alpha_b*cos(-alpha_r+4*pi/3)+z_l)/R_spool;

== matlab function UDP_Send_Poi_2021b_openloop_joystick_2023/modelGait1/RR ==
  data: alpha_r input; alpha_A output; alpha_b input; z_l input; alpha_B output; alpha_C output
function [alpha_A, alpha_B, alpha_C]= fcn(alpha_r, alpha_b, z_l)

L_disk = 0.02944;% Disk side length (m)
R_spool = 0.021;
R_w = L_disk/sqrt(3);

alpha_A = -(-R_w*alpha_b*cos(-alpha_r)+z_l)/R_spool;
alpha_B = -(-R_w*alpha_b*cos(-alpha_r+2*pi/3)+z_l)/R_spool;
alpha_C = -(-R_w*alpha_b*cos(-alpha_r+4*pi/3)+z_l)/R_spool;
